simulink model "Fig11"  (R2023b)
settings: Solver=ode1  StartTime=0.0  StopTime=600  FixedStep=1  RelTol=1e-3
settings Model: Creator=orlandojorquera  LastModifiedBy=evogel

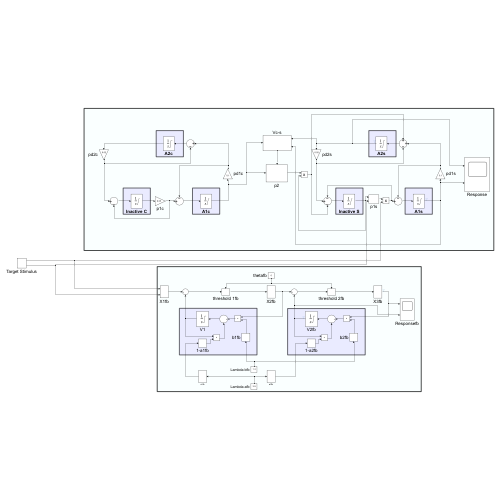
[thumbnail: Simulink's stored preview of the top-level diagram]
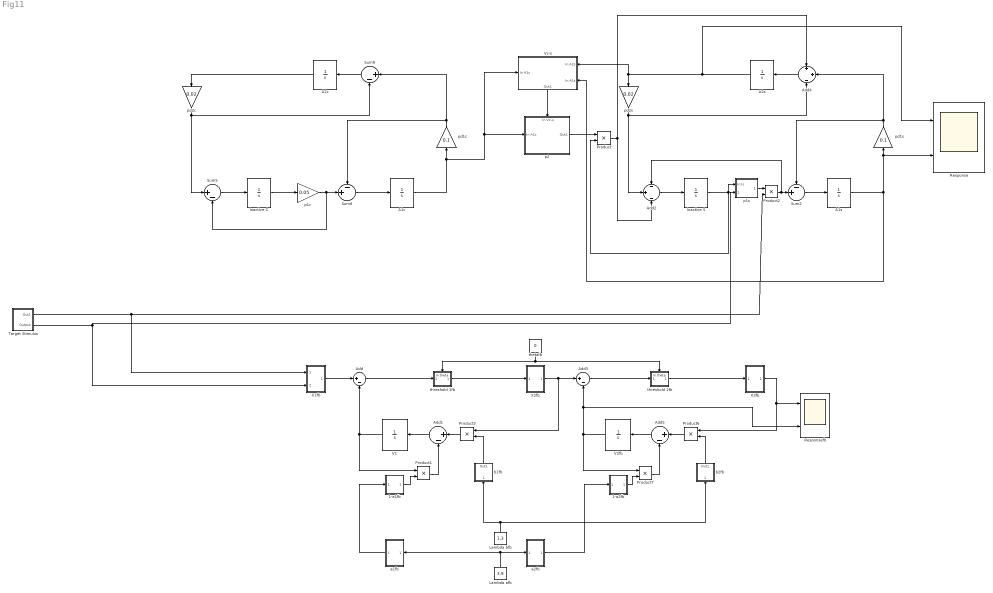
== system Fig11 ==
  1-a1fb : Subsystem
  1-a2fb : Subsystem
  A1c : Integrator  LimitOutput=on  LowerSaturationLimit=0
  A1s : Integrator  LimitOutput=on  LowerSaturationLimit=0
  A2c : Integrator  LimitOutput=on  LowerSaturationLimit=0
  A2s : Integrator  LimitOutput=on  LowerSaturationLimit=0
  Add{,1,3,5} (4 alike) : Sum  Inputs=|+-
  Add2 : Sum  Inputs=-|+|-
  Add4 : Sum  Inputs=+|+|-
  Inactive C : Integrator  InitialCondition=1  LimitOutput=on  LowerSaturationLimit=0
  Inactive S : Integrator  InitialCondition=1  LimitOutput=on  LowerSaturationLimit=0
  Lambda afb : Constant  Value=3.9
  Lambda bfb : Constant  Value=1.3
  Product{,1..3,6..7} (6 alike) : Product
  Response : Scope  NumInputPorts=2
  Responsefb : Scope  NumInputPorts=2
  Sum2 : Sum  Inputs=-+|
  Sum5 : Sum  Inputs=|+-
  Sum6 : Sum  Inputs=-+|
  Sum9 : Sum  Inputs=|+-
  Target Stimulus : Subsystem
  V1 : Integrator  LimitOutput=on
  V2fb : Integrator  LimitOutput=on
  Vc-s : Subsystem
      settings: PortSchema="{\"entries\":[{\"content\":{\"sides\":[{\"content\":{\"connectorIds\":[\"In1\"]},\"type\":\"ConnectorPlacement.EquallySpacedRectSide\",\"uuid\":\"b09f05bd-5603-47fe-a5ad-d7d6b3dc0c8e\"},{\"content\":{\"connectorIds\":[\"In2\",\"In3\"],\"side\":\"RIGHT\"},\"type\":\"ConnectorPlacement.EquallySpacedRectSide\",\"uuid\":\"d47795f3-6d8c-4c23-a554-34b772022c1b\"},{\"content\":{\"side\":\"TOP\"},\"type\":\"ConnectorPlacement.EquallySpacedRectSide\",\"uuid\":\"e48eddfd-d331-425c-b357-ebbea553df38\"},{\"content\":{\"connectorIds\":[\"Out1\"],\"side\":\"BOTTOM\"},\"type\":\"ConnectorPlacement.EquallySpacedRectSide\",\"uuid\":\"833a9385-f8e7-4f69-9c09-473a519a1ef8\"}]},\"type\":\"ConnectorPlacement.EquallySpacedConnector\",\"uuid\":\"43dd1673-4710-4827-90f7-71f5e88827f7\"}],\"packageUris\":[\"http://schema.mathworks.com/mf0/Connector/R2020b\"],\"version\":\"1.0\"}"
  X1fb : Subsystem
  X2fb : Subsystem
  X3fb : Subsystem
  a1fb : Subsystem
  a2fb : Subsystem
  b1fb : Subsystem
  b2fb : Subsystem
  p1c : Gain  Gain=0.05
  p1s : Subsystem
  p2 : Subsystem
      settings: PortSchema="{\"entries\":[{\"content\":{\"sides\":[{\"content\":{\"connectorIds\":[\"In1\"]},\"type\":\"ConnectorPlacement.EquallySpacedRectSide\",\"uuid\":\"e5de33b1-e289-4f06-b16e-f6995d6ff18d\"},{\"content\":{\"connectorIds\":[\"Out1\"],\"side\":\"RIGHT\"},\"type\":\"ConnectorPlacement.EquallySpacedRectSide\",\"uuid\":\"bf82b542-ee2f-4a07-ac72-0e3e2437644b\"},{\"content\":{\"connectorIds\":[\"In2\"],\"side\":\"TOP\"},\"type\":\"ConnectorPlacement.EquallySpacedRectSide\",\"uuid\":\"dbd75b9a-fc8b-4088-9d34-f07ad0492047\"}]},\"type\":\"ConnectorPlacement.EquallySpacedConnector\",\"uuid\":\"24fb73df-5fe4-4caa-a2a9-0eaf37dbdd75\"}],\"packageUris\":[\"http://schema.mathworks.com/mf0/Connector/R2020b\"],\"version\":\"1.0\"}"
  pd1c : Gain  Gain=0.1
  pd1s : Gain  Gain=0.1
  pd2c : Gain  Gain=0.02
  pd2s : Gain  Gain=0.02
  thetafb : Constant  Value=0
  threshold 1fb : Subsystem
      settings: PortSchema="{\"entries\":[{\"content\":{\"sides\":[{\"content\":{\"connectorIds\":[\"In1\"]},\"type\":\"ConnectorPlacement.EquallySpacedRectSide\",\"uuid\":\"df45c11a-cbfd-46b0-9931-ccf6bdc824b5\"},{\"content\":{\"connectorIds\":[\"Out1\"],\"side\":\"RIGHT\"},\"type\":\"ConnectorPlacement.EquallySpacedRectSide\",\"uuid\":\"7bdc14d3-84cb-4ad0-a730-e3b8f98cb716\"},{\"content\":{\"connectorIds\":[\"In2\"],\"side\":\"TOP\"},\"type\":\"ConnectorPlacement.EquallySpacedRectSide\",\"uuid\":\"6aa308ce-d9e8-4768-ab82-80fe1eba77b8\"}]},\"type\":\"ConnectorPlacement.EquallySpacedConnector\",\"uuid\":\"5c730a05-bfd2-4eaa-b46f-f4851af60a3b\"}],\"packageUris\":[\"http://schema.mathworks.com/mf0/Connector/R2020b\"],\"version\":\"1.0\"}"
  threshold 2fb : Subsystem
      settings: PortSchema="{\"entries\":[{\"content\":{\"sides\":[{\"content\":{\"connectorIds\":[\"In1\"]},\"type\":\"ConnectorPlacement.EquallySpacedRectSide\",\"uuid\":\"df45c11a-cbfd-46b0-9931-ccf6bdc824b5\"},{\"content\":{\"connectorIds\":[\"Out1\"],\"side\":\"RIGHT\"},\"type\":\"ConnectorPlacement.EquallySpacedRectSide\",\"uuid\":\"7bdc14d3-84cb-4ad0-a730-e3b8f98cb716\"},{\"content\":{\"connectorIds\":[\"In2\"],\"side\":\"TOP\"},\"type\":\"ConnectorPlacement.EquallySpacedRectSide\",\"uuid\":\"6aa308ce-d9e8-4768-ab82-80fe1eba77b8\"}]},\"type\":\"ConnectorPlacement.EquallySpacedConnector\",\"uuid\":\"5c730a05-bfd2-4eaa-b46f-f4851af60a3b\"}],\"packageUris\":[\"http://schema.mathworks.com/mf0/Connector/R2020b\"],\"version\":\"1.0\"}"
  wires:
  Inactive C/1 -> p1c/1
  Sum5/1 -> Inactive C/1
  p1c/1 -> Sum6/2, Sum5/2
  pd1c/1 -> Sum9/1, Sum6/1
  Sum6/1 -> A1c/1
  A1c/1 -> Vc-s/1(In A1c), p2/1(In A1c), pd1c/1
  Sum9/1 -> A2c/1
  A2c/1 -> pd2c/1
  pd2c/1 -> Sum5/1, Sum9/2
  Vc-s/1(Out1) -> p2/2(In Vc-s)
  pd2s/1 -> Add4/3, Add2/2
  A2s/1 -> Response/1, pd2s/1, Vc-s/2(In A2s)
  Add4/1 -> A2s/1
  A1s/1 -> Response/2, pd1s/1, Vc-s/3(In A1s)
  Sum2/1 -> A1s/1
  pd1s/1 -> Add4/2, Sum2/1
  Add2/1 -> Inactive S/1
  Inactive S/1 -> p1s/1(In Is), Product/2
  Product2/1 -> Add2/1, Sum2/2
  p1s/1(Output) -> Product2/1
  p2/1(Out1) -> Product/1
  Product/1 -> Add2/3, Add4/1
  1-a1fb/1(Out1) -> Product1/2
  Add3/1 -> threshold 2fb/1(In X2 - V2)
  Add/1 -> threshold 1fb/1(In X1 - V1)
  a1fb/1(Out1) -> 1-a1fb/1(In a1)
  X2fb/1(Out1) -> Product3/1, Add3/1
  1-a2fb/1(Out1) -> Product7/2
  X3fb/1(Out1) -> Product6/1, Responsefb/1
  V1/1 -> Product1/1, Add/2
  Add5/1 -> V2fb/1
  Product1/1 -> Add1/2
  V2fb/1 -> Add3/2, Responsefb/2, Product7/1
  threshold 2fb/1(Out1) -> X3fb/1(In1)
  Lambda bfb/1 -> b1fb/1(In lambda_b), b2fb/1(In lambda_b)
  Lambda afb/1 -> a1fb/1(In lambda_a), a2fb/1(In lambda_a)
  Add1/1 -> V1/1
  b2fb/1(Out1) -> Product6/2
  thetafb/1 -> threshold 1fb/2(In theta), threshold 2fb/2(In theta)
  a2fb/1(Out1) -> 1-a2fb/1(In a2)
  Product6/1 -> Add5/1
  b1fb/1(Out1) -> Product3/2
  threshold 1fb/1(Out1) -> X2fb/1(In1)
  Product3/1 -> Add1/1
  X1fb/1(Output) -> Add/1
  Product7/1 -> Add5/2
  Target Stimulus/1(Out1) -> Product2/2, X1fb/1(In Stimulus)
  Target Stimulus/2(Output) -> p1s/2(In Intensity), X1fb/2(In Intensity)

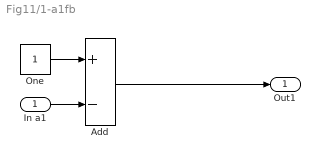
== system Fig11/1-a1fb ==
  In a1 : Inport
  Add : Sum  Inputs=+-
  One : Constant  OutDataTypeStr=Inherit: Inherit via back propagation
  Out1 : Outport
  wires:
  One/1 -> Add/1
  Add/1 -> Out1/1
  In a1/1 -> Add/2

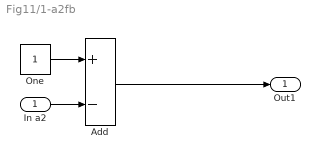
== system Fig11/1-a2fb ==
  In a2 : Inport
  Add : Sum  Inputs=+-
  One : Constant  OutDataTypeStr=Inherit: Inherit via back propagation
  Out1 : Outport
  wires:
  In a2/1 -> Add/2
  Add/1 -> Out1/1
  One/1 -> Add/1

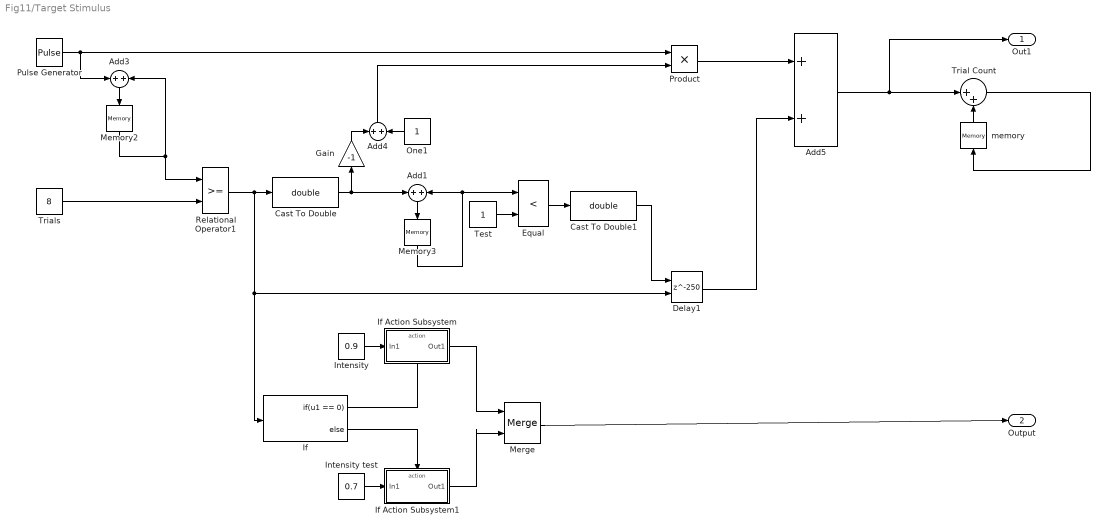
== system Fig11/Target Stimulus ==
  Add{1,3..5} (4 alike) : Sum
  Cast To Double : DataTypeConversion  OutDataTypeStr=double  SaturateOnIntegerOverflow=off  RndMeth=Floor
  Cast To Double1 : DataTypeConversion  OutDataTypeStr=double  SaturateOnIntegerOverflow=off  RndMeth=Floor
  Delay1 : Delay  DelayLength=250  ShowEnablePort=on
      settings: InputPortMap=u0,e6
  Equal : RelationalOperator  Operator=<  OutDataTypeStr=boolean  RndMeth=Simplest  InputSameDT=off
  Gain : Gain  Gain=-1
  If : If  IfExpression=u1 == 0
  If Action Subsystem : Subsystem  TreatAsAtomicUnit=on
  If Action Subsystem1 : Subsystem  TreatAsAtomicUnit=on
  Intensity : Constant  Value=0.9
  Intensity test : Constant  Value=0.7
  Memory2 : Memory
  Memory3 : Memory
  Merge : Merge
  One1 : Constant  OutDataTypeStr=Inherit: Inherit via back propagation
  Product : Product
  Pulse Generator : DiscretePulseGenerator  Period=60  PhaseDelay=30
  Relational Operator1 : RelationalOperator  OutDataTypeStr=boolean  RndMeth=Simplest  InputSameDT=off
  Test : Constant  OutDataTypeStr=Inherit: Inherit via back propagation
  Trial Count : Sum  Inputs=|++
  Trials : Constant  Value=8
  memory : Memory
  Out1 : Outport
  Output : Outport  Port=2
  wires:
  Pulse Generator/1 -> Add3/1, Product/1
  Add3/1 -> Memory2/1
  Memory2/1 -> Relational Operator1/1, Add3/2
  Trials/1 -> Relational Operator1/2
  Relational Operator1/1 -> Cast To Double/1, Delay1/2, If/1
  Cast To Double/1 -> Gain/1, Add1/1
  Add1/1 -> Memory3/1
  Memory3/1 -> Add1/2, Equal/1
  Test/1 -> Equal/2
  Equal/1 -> Cast To Double1/1
  Gain/1 -> Add4/1
  One1/1 -> Add4/2
  Add4/1 -> Product/2
  Cast To Double1/1 -> Delay1/1
  Product/1 -> Add5/1
  Delay1/1 -> Add5/2
  Add5/1 -> Trial Count/1, Out1/1
  If/1 -> If Action Subsystem/Action
  If/2 -> If Action Subsystem1/Action
  Intensity/1 -> If Action Subsystem/1(In1)
  Intensity test/1 -> If Action Subsystem1/1(In1)
  If Action Subsystem/1(Out1) -> Merge/1
  If Action Subsystem1/1(Out1) -> Merge/2
  Merge/1 -> Output/1
  Trial Count/1 -> memory/1
  memory/1 -> Trial Count/2

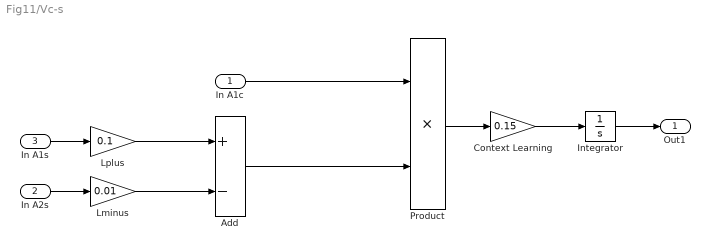
== system Fig11/Vc-s ==
  In A1c : Inport
  In A2s : Inport  Port=2
  In A1s : Inport  Port=3
  Add : Sum  Inputs=+-
  Context Learning : Gain  Gain=0.15
  Integrator : Integrator  LimitOutput=on  LowerSaturationLimit=0
  Lminus : Gain  Gain=0.01
  Lplus : Gain  Gain=0.1
  Product : Product
  Out1 : Outport
  wires:
  In A1s/1 -> Lplus/1
  In A2s/1 -> Lminus/1
  In A1c/1 -> Product/1
  Product/1 -> Context Learning/1
  Context Learning/1 -> Integrator/1
  Add/1 -> Product/2
  Lplus/1 -> Add/1
  Lminus/1 -> Add/2
  Integrator/1 -> Out1/1

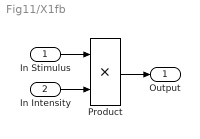
== system Fig11/X1fb ==
  In Stimulus : Inport
  In Intensity : Inport  Port=2
  Product : Product
  Output : Outport
  wires:
  In Stimulus/1 -> Product/1
  Product/1 -> Output/1
  In Intensity/1 -> Product/2

== system Fig11/X2fb ==
  In1 : Inport
  Out1 : Outport
  wires:
  In1/1 -> Out1/1

== system Fig11/X3fb ==
  In1 : Inport
  Out1 : Outport
  wires:
  In1/1 -> Out1/1

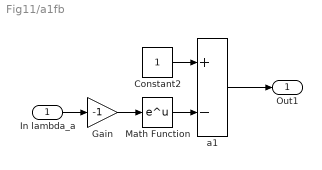
== system Fig11/a1fb ==
  In lambda_a : Inport
  Constant2 : Constant
  Gain : Gain  Gain=-1
  Math Function : Math
  a1 : Sum  Inputs=+-
  Out1 : Outport
  wires:
  Math Function/1 -> a1/2
  Gain/1 -> Math Function/1
  Constant2/1 -> a1/1
  In lambda_a/1 -> Gain/1
  a1/1 -> Out1/1

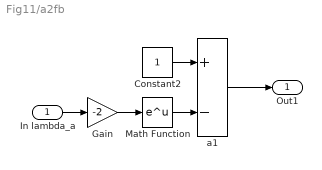
== system Fig11/a2fb ==
  In lambda_a : Inport
  Constant2 : Constant
  Gain : Gain  Gain=-2
  Math Function : Math
  a1 : Sum  Inputs=+-
  Out1 : Outport
  wires:
  a1/1 -> Out1/1
  In lambda_a/1 -> Gain/1
  Constant2/1 -> a1/1
  Gain/1 -> Math Function/1
  Math Function/1 -> a1/2

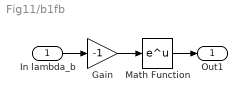
== system Fig11/b1fb ==
  In lambda_b : Inport
  Gain : Gain  Gain=-1
  Math Function : Math
  Out1 : Outport
  wires:
  Math Function/1 -> Out1/1
  In lambda_b/1 -> Gain/1
  Gain/1 -> Math Function/1

== system Fig11/b2fb ==
  In lambda_b : Inport
  Gain : Gain  Gain=-2
  Math Function : Math
  Out1 : Outport
  wires:
  Gain/1 -> Math Function/1
  In lambda_b/1 -> Gain/1
  Math Function/1 -> Out1/1

== system Fig11/p1s ==
  In Is : Inport
  In Intensity : Inport  Port=2
  Product : Product
  Output : Outport
  wires:
  In Intensity/1 -> Product/2
  In Is/1 -> Product/1
  Product/1 -> Output/1

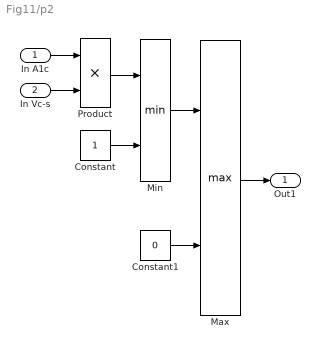
== system Fig11/p2 ==
  In A1c : Inport
  In Vc-s : Inport  Port=2
  Constant : Constant
  Constant1 : Constant  Value=0
  Max : MinMax  Function=max  Inputs=2
  Min : MinMax  Inputs=2
  Product : Product
  Out1 : Outport
  wires:
  In Vc-s/1 -> Product/2
  In A1c/1 -> Product/1
  Product/1 -> Min/1
  Constant/1 -> Min/2
  Min/1 -> Max/1
  Constant1/1 -> Max/2
  Max/1 -> Out1/1

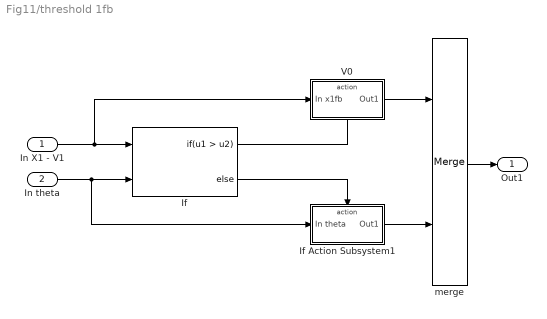
== system Fig11/threshold 1fb ==
  In X1 - V1 : Inport
  In theta : Inport  Port=2
  If : If  NumInputs=2  IfExpression=u1 > u2
  If Action Subsystem1 : Subsystem  TreatAsAtomicUnit=on
  V0 : Subsystem  TreatAsAtomicUnit=on
  merge : Merge
  Out1 : Outport
  wires:
  V0/1(Out1) -> merge/1
  merge/1 -> Out1/1
  If Action Subsystem1/1(Out1) -> merge/2
  In theta/1 -> If Action Subsystem1/1(In theta), If/2
  In X1 - V1/1 -> V0/1(In x1fb), If/1
  If/1 -> V0/Action
  If/2 -> If Action Subsystem1/Action

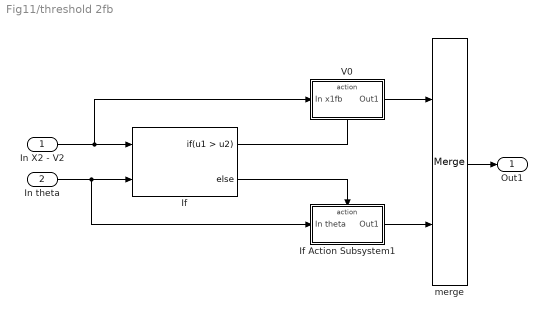
== system Fig11/threshold 2fb ==
  In X2 - V2 : Inport
  In theta : Inport  Port=2
  If : If  NumInputs=2  IfExpression=u1 > u2
  If Action Subsystem1 : Subsystem  TreatAsAtomicUnit=on
  V0 : Subsystem  TreatAsAtomicUnit=on
  merge : Merge
  Out1 : Outport
  wires:
  If/2 -> If Action Subsystem1/Action
  If/1 -> V0/Action
  In X2 - V2/1 -> If/1, V0/1(In x1fb)
  In theta/1 -> If/2, If Action Subsystem1/1(In theta)
  If Action Subsystem1/1(Out1) -> merge/2
  merge/1 -> Out1/1
  V0/1(Out1) -> merge/1

== system Fig11/Target Stimulus/If Action Subsystem ==
  In1 : Inport
  Action Port : ActionPort  ActionPortLabel=if(u1 == 0)
  Out1 : Outport
  wires:
  In1/1 -> Out1/1

== system Fig11/Target Stimulus/If Action Subsystem1 ==
  In1 : Inport
  Action Port : ActionPort  ActionPortLabel=else
  Out1 : Outport
  wires:
  In1/1 -> Out1/1

== system Fig11/threshold 1fb/If Action Subsystem1 ==
  In theta : Inport
  Action Port : ActionPort  ActionPortLabel=else
  Out1 : Outport
  wires:
  In theta/1 -> Out1/1

== system Fig11/threshold 1fb/V0 ==
  In x1fb : Inport
  Action Port : ActionPort  ActionPortLabel=if(u1 > u2)
  Out1 : Outport
  wires:
  In x1fb/1 -> Out1/1

== system Fig11/threshold 2fb/If Action Subsystem1 ==
  In theta : Inport
  Action Port : ActionPort  ActionPortLabel=else
  Out1 : Outport
  wires:
  In theta/1 -> Out1/1

== system Fig11/threshold 2fb/V0 ==
  In x1fb : Inport
  Action Port : ActionPort  ActionPortLabel=if(u1 > u2)
  Out1 : Outport
  wires:
  In x1fb/1 -> Out1/1
